simulink model "noload_shortcircuit_tests"  (R2016b)
settings: Solver=ode23t  StartTime=0.0  StopTime=1  MaxStep=1e-4  RelTol=1e-4  AbsTol=1e-4  EnableMultiTasking=on
InitFcn:
  | param
values from neighbouring files (symbols this model uses):
  P = 6    [param.m]
  R = 0.37    [param.m]
libraries: fl_lib x6, nesl_utility x4, pe_lib x3, ThreePhaseExamples_lib x1
Description:
  | Three-Phase Custom PMSM
  | 
  | This example shows a custom Simscape(TM) implementation of
  | a Permanent Magnet Synchronous Machine (PMSM). To view the
  | PMSM source code, double-click on the motor block and then
  | click on the hyperlink 'Source code'. This test circuit shows the
  | PMSM being used as a generator, the rectifier block converting
  | the induced AC back EMFs to a DC voltage which is in turn
  | applied to a resistive load.
  | 
  | 
  | 
  | Copyright 2008-2016 The MathWorks, Inc.
settings Model: Creator=MathWorks  LastModifiedBy=Philipp
settings DataIOCC: LimitDataPoints=on  SaveFormat=Array
settings OptimizationCC: LifeSpan=inf
settings DebuggingCC: UnderspecifiedInitializationDetection=Classic  MergeDetectMultiDrivingBlocksExec=none  SFUnexpectedBacktrackingDiag=warning  SFNoUnconditionalDefaultTransitionDiag=warning  SFExecutionAtInitializationDiag=none
settings HardwareCC: ProdBitPerPointer=32  ProdBitPerSizeT=32  ProdBitPerPtrDiffT=32  ProdLargestAtomicFloat=None  ProdIntDivRoundTo=Undefined  ProdEndianess=Unspecified  ProdWordSize=32  ProdHWDeviceType=32-bit Generic
settings ModelReferenceCC: PropagateSignalLabelsOutOfModel=off
settings GRTTargetCC: TargetLangStandard=C89/C90 (ANSI)  GeneratePreprocessorConditionals=Disable all
settings ConfigComp: CovMetricSettings=dw  CovHtmlReporting=on  CovSaveCumulativeToWorkspaceVar=on  CovSaveSingleToWorkspaceVar=on  CovExternalEMLEnable=off  CovSFcnEnable=off
settings SimscapeCC: SimscapeLogDataHistory=50000

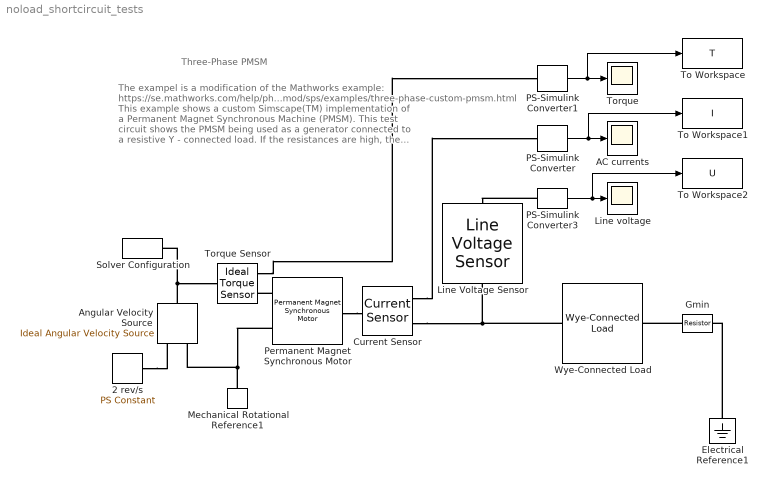
== system noload_shortcircuit_tests ==
  note: The exampel is a modification of the Mathworks example: https://se.mathworks.com/help/physmod/sps/examples/three-phase-custom-pmsm.html
      | This example shows a custom Simscape(TM) implementation of a Permanent Magnet Synchronous Machine (PMSM).
      | This test circuit shows the PMSM being used as a generator connected to a resistive Y - connected load.
      | If the resistances are high, the currents will be zero (low) and the voltages between the terminals is the induced voltages (no load voltage).
      | If the resistances are low, the machine will be short circuited ( almost).
  note: Three-Phase PMSM
  2 rev/s : fl_lib/Physical Signals/Sources/PS Constant  constant=w_mech
  AC currents : Scope
  Angular Velocity Source : fl_lib/Mechanical/Mechanical Sources/Ideal Angular Velocity Source
  Current Sensor : pe_lib/Sensors/Current Sensor
  Electrical Reference1 : fl_lib/Electrical/Electrical Elements/Electrical Reference
  Gmin : fl_lib/Electrical/Electrical Elements/Resistor  R=1e9 Ohm  i_specify=off  i_priority=High  i=0 A  v_specify=off  v_priority=High  v=0 V
  Line Voltage Sensor : pe_lib/Sensors/Line Voltage Sensor
  Line voltage : Scope
  Mechanical Rotational Reference1 : fl_lib/Mechanical/Rotational Elements/Mechanical Rotational Reference
  PS-Simulink Converter : nesl_utility/PS-Simulink Converter  PhysicalDomain=network_engine_domain  SubClassName=ps_output  LeftPortType=input  RightPortType=output  PseudoPeriodic=off  Frequencies=[]  Unit=A  AffineConversion=off
  PS-Simulink Converter1 : nesl_utility/PS-Simulink Converter  PhysicalDomain=network_engine_domain  SubClassName=ps_output  LeftPortType=input  RightPortType=output  PseudoPeriodic=off  Frequencies=[]  Unit=N*m  AffineConversion=off
  PS-Simulink Converter3 : nesl_utility/PS-Simulink Converter  PhysicalDomain=network_engine_domain  SubClassName=ps_output  LeftPortType=input  RightPortType=output  PseudoPeriodic=off  Frequencies=[]  Unit=V  AffineConversion=off
  Permanent Magnet Synchronous Motor : ThreePhaseExamples_lib/Permanent Magnet Synchronous Motor  nPolePairs=P/2  pm_flux_linkage=psi_m N*m/A  Ld=L H  Lq=L H  Rs=R/2 Ohm  wNominal=0 rad/s  angular_position_diff_specify=off  angular_position_diff_priority=None  angular_position_diff=0 rad  i_d_specify=off  i_d_priority=High  i_d=0 A  i_q_specify=off  i_q_priority=High  i_q=0 A
  Solver Configuration : nesl_utility/Solver Configuration  PhysicalDomain=network_engine_domain  SubClassName=solver  LeftPortType=input  RightPortType=generic  Accelerate=off  Tones=[]  Harmonics=[]  SimulateNoise=off  Profile=off  UseLocalSampling=off  EnableSwitchedLinearOptims=on  FrequencyDomain=off  UseCCode=off  RelTol=0.001  AbsTol=1e-06  MinStep=1e-09  ToWorkspace=off  RevertToSquareIcSolve=off  NumHomotopyIterations=100  PhasorMode=off  PhasorModeNumHarmonics=1  OverrideAbsTol=off  DoDC=off  ResidualTolerance=1e-9  UseLocalSolver=on  LocalSolverChoice=NE_BACKWARD_EULER_ADVANCER  LocalSolverSampleTime=1e-5  DoFixedCost=on  MaxNonlinIter=3  MaxModeIter=2  LinearAlgebra=Sparse  DelaysMemoryBudget=1024  AutomaticFiltering=on  FilteringTimeConstant=0.001
  To Workspace : ToWorkspace  VariableName=T  SaveFormat=Timeseries  SampleTime=-1
  To Workspace1 : ToWorkspace  VariableName=I  SaveFormat=Timeseries  SampleTime=-1
  To Workspace2 : ToWorkspace  VariableName=U  SaveFormat=Timeseries  SampleTime=-1
  Torque : Scope
  Torque Sensor : fl_lib/Mechanical/Mechanical Sensors/Ideal Torque Sensor
  Wye-Connected Load : pe_lib/Passive Devices/Wye-Connected Load  parameterization=1  component_structure=1  component_structure_PQ=1  R=1e3 Ohm  L=0.001 H  C=1e-6 F  IL0=[ 0 0 0 ] A  VC0=[ 0 0 0 ] V  R_parasitic=1e-6 Ohm  G_parasitic=1e-6 1/Ohm  VRated=2.4e+4 V  FRated=60 Hz  P=1000 W  Qpos=100 V*A  Qneg=-100 V*A  Vmag0=2.4e+4 V  Vang0=0 deg  Freq0=60 Hz  R_parasitic_PQ=1e-6 Ohm  G_parasitic_PQ=1e-6 1/Ohm
  wires:
  PS-Simulink Converter/1 -> To Workspace1/1, AC currents/1
  PS-Simulink Converter1/1 -> To Workspace/1, Torque/1
  PS-Simulink Converter3/1 -> To Workspace2/1, Line voltage/1
  connections:
  Mechanical Rotational Reference1/LConn1 -- Permanent Magnet Synchronous Motor/RConn2 -- Angular Velocity Source/RConn2
  Permanent Magnet Synchronous Motor/LConn1 -- Current Sensor/LConn1
  Current Sensor/RConn1 -- PS-Simulink Converter/LConn1
  Permanent Magnet Synchronous Motor/RConn1 -- Torque Sensor/RConn1
  Torque Sensor/RConn2 -- PS-Simulink Converter1/LConn1
  2 rev/s/RConn1 -- Angular Velocity Source/RConn1
  Angular Velocity Source/LConn1 -- Solver Configuration/RConn1 -- Torque Sensor/LConn1
  Current Sensor/RConn2 -- Line Voltage Sensor/LConn1 -- Wye-Connected Load/LConn1
  Electrical Reference1/LConn1 -- Gmin/LConn1
  PS-Simulink Converter3/LConn1 -- Line Voltage Sensor/RConn1
  Gmin/RConn1 -- Wye-Connected Load/RConn1
